simulink library "momentumVelocityControl_lib"  (R2020b)
settings: Solver=VariableStepAuto  StartTime=0.0  StopTime=10.0  RelTol=1e-3
undefined symbols (not defined in the file): bVectorConstraints, Config, ConstraintsMatrix, ROBOT_DOF, Sat
settings Model: Creator=csartore  LastModifiedBy=csartore

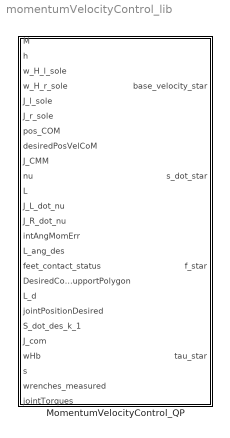
== system momentumVelocityControl_lib ==
  MomentumVelocityControl_QP : Subsystem

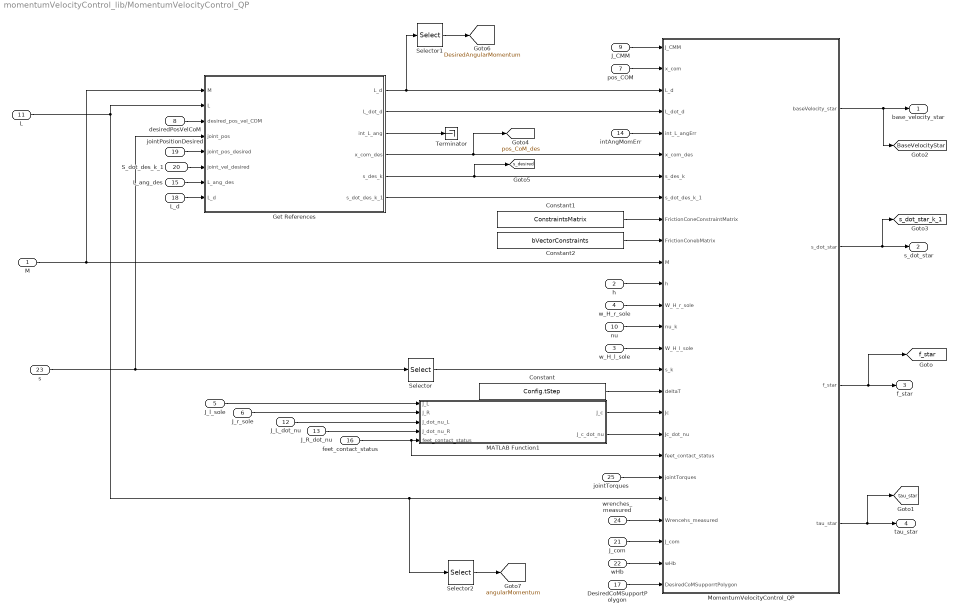
== system momentumVelocityControl_lib/MomentumVelocityControl_QP ==
  M : Inport
  h : Inport  Port=2
  w_H_l_sole : Inport  Port=3
  w_H_r_sole : Inport  Port=4
  J_l_sole : Inport  Port=5
  J_r_sole : Inport  Port=6
  pos_COM : Inport  Port=7
  desiredPosVelCoM : Inport  Port=8
  J_CMM : Inport  Port=9
  nu : Inport  Port=10
  L : Inport  Port=11
  J_L_dot_nu : Inport  Port=12
  J_R_dot_nu : Inport  Port=13
  intAngMomErr : Inport  Port=14
  L_ang_des : Inport  Port=15
  feet_contact_status : Inport  Port=16
  DesiredCoMSupportPolygon : Inport  Port=17
  L_d : Inport  Port=18
  jointPositionDesired : Inport  Port=19
  S_dot_des_k_1 : Inport  Port=20
  J_com : Inport  Port=21
  wHb : Inport  Port=22
  s : Inport  Port=23
  wrenches_measured : Inport  Port=24
  jointTorques : Inport  Port=25
  Constant : Constant  Value=Config.tStep
  Constant1 : Constant  Value=ConstraintsMatrix
  Constant2 : Constant  Value=bVectorConstraints
  Get References : MATLAB Function  TreatAsAtomicUnit=on
  MATLAB Function1 : MATLAB Function  TreatAsAtomicUnit=on
  MomentumVelocityControl_QP : Subsystem
  Selector : Selector  InputPortWidth=ROBOT_DOF  IndexOptions=Index vector (dialog)  Indices=[1:ROBOT_DOF]  OutputSizes=1
  Selector1 : Selector  InputPortWidth=6  IndexOptions=Index vector (dialog)  Indices=[4:6]  OutputSizes=1
  Selector2 : Selector  InputPortWidth=6  IndexOptions=Index vector (dialog)  Indices=[4:6]  OutputSizes=1
  Terminator : Terminator
  base_velocity_star : Outport
  s_dot_star : Outport  Port=2
  f_star : Outport  Port=3
  tau_star : Outport  Port=4
  tag scope: BaseVelocityStar=global, DesiredAngularMomentum=global, angularMomentum=global, f_star=global, pos_CoM_des=global, s_desired=global, s_dot_star_k_1=global, tau_star=global
  wires:
  DesiredCoMSupportPolygon/1 -> MomentumVelocityControl_QP/26(DesiredCoMSupporrtPolygon)
  Get References/6(s_dot_des_k_1) -> MomentumVelocityControl_QP/8(s_dot_des_k_1)
  Selector2/1 -> [angularMomentum]
  Selector1/1 -> [DesiredAngularMomentum]
  Selector/1 -> MomentumVelocityControl_QP/16(s_k)
  h/1 -> MomentumVelocityControl_QP/12(h)
  L/1 -> MomentumVelocityControl_QP/22(L), Selector2/1, Get References/2(L)
  J_CMM/1 -> MomentumVelocityControl_QP/1(J_CMM)
  MATLAB Function1/2(J_c_dot_nu) -> MomentumVelocityControl_QP/19(Jc_dot_nu)
  intAngMomErr/1 -> MomentumVelocityControl_QP/5(int_L_angErr)
  MomentumVelocityControl_QP/2(s_dot_star) -> [s_dot_star_k_1], s_dot_star/1
  MomentumVelocityControl_QP/1(baseVelocity_star) -> [BaseVelocityStar], base_velocity_star/1
  MATLAB Function1/1(J_c) -> MomentumVelocityControl_QP/18(Jc)
  nu/1 -> MomentumVelocityControl_QP/14(nu_k)
  feet_contact_status/1 -> MATLAB Function1/5(feet_contact_status), MomentumVelocityControl_QP/20(feet_contact_status)
  MomentumVelocityControl_QP/4(tau_star) -> [tau_star], tau_star/1
  L_ang_des/1 -> Get References/7(L_ang_des)
  Get References/5(s_des_k) -> MomentumVelocityControl_QP/7(s_des_k), [s_desired]
  pos_COM/1 -> MomentumVelocityControl_QP/2(x_com)
  w_H_r_sole/1 -> MomentumVelocityControl_QP/13(W_H_r_sole)
  w_H_l_sole/1 -> MomentumVelocityControl_QP/15(W_H_l_sole)
  J_r_sole/1 -> MATLAB Function1/2(J_R)
  Get References/2(L_dot_d) -> MomentumVelocityControl_QP/4(L_dot_d)
  jointPositionDesired/1 -> Get References/5(joint_pos_desired)
  J_R_dot_nu/1 -> MATLAB Function1/4(J_dot_nu_R)
  s/1 -> Selector/1, Get References/4(joint_pos)
  jointTorques/1 -> MomentumVelocityControl_QP/21(jointTorques)
  J_L_dot_nu/1 -> MATLAB Function1/3(J_dot_nu_L)
  wHb/1 -> MomentumVelocityControl_QP/25(wHb)
  wrenches_measured/1 -> MomentumVelocityControl_QP/23(Wrencehs_measured)
  Constant1/1 -> MomentumVelocityControl_QP/9(FrictionConeConstraintMatrix)
  M/1 -> MomentumVelocityControl_QP/11(M), Get References/1(M)
  MomentumVelocityControl_QP/3(f_star) -> [f_star], f_star/1
  Constant/1 -> MomentumVelocityControl_QP/17("deltaT ")
  Constant2/1 -> MomentumVelocityControl_QP/10(FrictionConebMatrix)
  Get References/4(x_com_des) -> MomentumVelocityControl_QP/6(x_com_des), [pos_CoM_des]
  J_l_sole/1 -> MATLAB Function1/1(J_L)
  Get References/1(L_d) -> Selector1/1, MomentumVelocityControl_QP/3(L_d)
  Get References/3(int_L_ang) -> Terminator/1
  J_com/1 -> MomentumVelocityControl_QP/24(J_com)
  desiredPosVelCoM/1 -> Get References/3(desired_pos_vel_COM)
  L_d/1 -> Get References/8("L_d ")
  S_dot_des_k_1/1 -> Get References/6(joint_vel_desired)

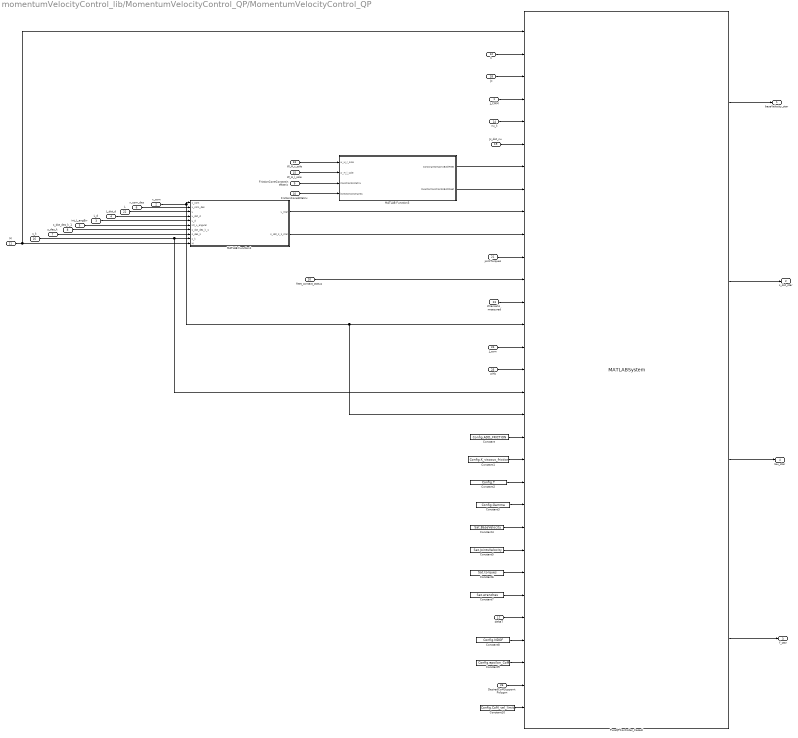
== system momentumVelocityControl_lib/MomentumVelocityControl_QP/MomentumVelocityControl_QP ==
  J_CMM : Inport
  x_com : Inport  Port=2
  L_d : Inport  Port=3
  L_dot_d : Inport  Port=4
  int_L_angErr : Inport  Port=5
  x_com_des : Inport  Port=6
  s_des_k : Inport  Port=7
  s_dot_des_k_1 : Inport  Port=8
  FrictionConeConstraintMatrix : Inport  Port=9
  FrictionConebMatrix : Inport  Port=10
  M : Inport  Port=11
  h : Inport  Port=12
  W_H_r_sole : Inport  Port=13
  nu_k : Inport  Port=14
  W_H_l_sole : Inport  Port=15
  s_k : Inport  Port=16
  "deltaT " : Inport  Port=17
  Jc : Inport  Port=18
  Jc_dot_nu : Inport  Port=19
  feet_contact_status : Inport  Port=20
  jointTorques : Inport  Port=21
  L : Inport  Port=22
  Wrencehs_measured : Inport  Port=23
  J_com : Inport  Port=24
  wHb : Inport  Port=25
  DesiredCoMSupporrtPolygon : Inport  Port=26
  Constant : Constant  Value=Config.ADD_FRICTION
  Constant1 : Constant  Value=Config.K_viscous_friction
  Constant10 : Constant  Value=Config.CoM_vel_limits  VectorParams1D=off
  Constant2 : Constant  Value=Config.T
  Constant3 : Constant  Value=Config.Gamma
  Constant4 : Constant  Value=Sat.BaseVelocity  VectorParams1D=off
  Constant5 : Constant  Value=Sat.JointsVelocity  VectorParams1D=off
  Constant6 : Constant  Value=Sat.torques  VectorParams1D=off
  Constant7 : Constant  Value=Sat.wrenches  VectorParams1D=off
  Constant8 : Constant  Value=Config.NDOF  VectorParams1D=off
  Constant9 : Constant  Value=Config.epsilon_CoM  VectorParams1D=off
  MATLAB Function1 : MATLAB Function  TreatAsAtomicUnit=on
  MATLAB Function3 : MATLAB Function  TreatAsAtomicUnit=on
  PureQPController_Casadi : MATLABSystem  System=casadi_block  SimulateUsing=Interpreted execution
      mask Type: casadi_block
      mask Display:
      | disp('casadi_block');
      | port_label('input',1,'M');
      | port_label('input',2,'h');
      | port_label('input',3,'Jc');
      | port_label('input',4,'Jcmm');
      | port_label('input',5,'nu_k');
      | port_label('input',6,'Jc_dot_nu');
      | port_label('input',7,'C_friction');
      | port_label('input',8,'b_friction');
      | port_label('input',9,'H_star');
      | port_label('input',10,'s_dot_star');
      | port_label('input',11,'tau_meas');
      | port_label('input',12,'contact_status');
      | port_label('input',13,'f_meas');
      | port_label('input',14,'x_com');
      | port_label('input',15,'J_com');
      | port_label('input',16,'w_H_b');
      | port_label('input',17,'s');
      | port_label('input',18,'CoM_measured');
      | port_label('input',19,'ADD_FRICTION');
      | port_label('input',20,'K_viscous_friction');
      | port_label('input',21,'T');
      | port_label('input',22,'Gamma');
      | port_label('input',23,'baseVelocitySat');
      | port_label('input',24,'jointsVelocitySat');
      | port_label('input',25,'torqueSat');
      | port_label('input',26,'wrenchesSat');
      | port_label('input',27,'tStep');
      | port_label('input',28,'NDOF');
      | port_label('input',29,'epsilon_CoM');
      | port_label('input',30,'CoM_limits');
      | port_label('input',31,'CoM_vel_limits');
      | port_label('output',1,'v_b_star');
      | port_label('output',2,'s_dot_k_1_star');
      | port_label('output',3,'tau_star');
      | port_label('output',4,'f_star');
  baseVelocity_star : Outport
  s_dot_star : Outport  Port=2
  f_star : Outport  Port=3
  tau_star : Outport  Port=4
  wires:
  PureQPController_Casadi/4 -> f_star/1
  PureQPController_Casadi/1 -> baseVelocity_star/1
  PureQPController_Casadi/3 -> tau_star/1
  PureQPController_Casadi/2 -> s_dot_star/1
  Constant10/1 -> PureQPController_Casadi/31
  DesiredCoMSupporrtPolygon/1 -> PureQPController_Casadi/30
  Constant9/1 -> PureQPController_Casadi/29
  Constant8/1 -> PureQPController_Casadi/28
  "deltaT "/1 -> PureQPController_Casadi/27
  Constant7/1 -> PureQPController_Casadi/26
  Constant6/1 -> PureQPController_Casadi/25
  Constant5/1 -> PureQPController_Casadi/24
  Constant4/1 -> PureQPController_Casadi/23
  Constant3/1 -> PureQPController_Casadi/22
  Constant2/1 -> PureQPController_Casadi/21
  Constant1/1 -> PureQPController_Casadi/20
  Constant/1 -> PureQPController_Casadi/19
  jointTorques/1 -> PureQPController_Casadi/11
  MATLAB Function1/1(L_star) -> PureQPController_Casadi/9
  MATLAB Function1/2(s_dot_k_1_star) -> PureQPController_Casadi/10
  MATLAB Function3/1(ConstraintsMatrixBothFeet) -> PureQPController_Casadi/7
  MATLAB Function3/2(bVectorConstraintsBothFeet) -> PureQPController_Casadi/8
  W_H_r_sole/1 -> MATLAB Function3/1(w_H_r_sole)
  W_H_l_sole/1 -> MATLAB Function3/2(w_H_l_sole)
  x_com/1 -> MATLAB Function1/1(x_com), PureQPController_Casadi/14, PureQPController_Casadi/18
  x_com_des/1 -> MATLAB Function1/2(x_com_des)
  L/1 -> MATLAB Function1/3(L)
  L_dot_d/1 -> MATLAB Function1/4(L_dot_d)
  L_d/1 -> MATLAB Function1/5(L_d)
  int_L_angErr/1 -> MATLAB Function1/6(int_L_angular)
  s_des_k/1 -> MATLAB Function1/8(s_des_k)
  s_dot_des_k_1/1 -> MATLAB Function1/7(s_dot_des_k_1)
  M/1 -> MATLAB Function1/10(M), PureQPController_Casadi/1
  feet_contact_status/1 -> PureQPController_Casadi/12
  Jc/1 -> PureQPController_Casadi/3
  J_CMM/1 -> PureQPController_Casadi/4
  nu_k/1 -> PureQPController_Casadi/5
  Jc_dot_nu/1 -> PureQPController_Casadi/6
  h/1 -> PureQPController_Casadi/2
  FrictionConeConstraintMatrix/1 -> MATLAB Function3/3(ConstraintsMatrix)
  FrictionConebMatrix/1 -> MATLAB Function3/4(bVectorConstraints)
  Wrencehs_measured/1 -> PureQPController_Casadi/13
  J_com/1 -> PureQPController_Casadi/15
  wHb/1 -> PureQPController_Casadi/16
  s_k/1 -> PureQPController_Casadi/17, MATLAB Function1/9(s_k)

== matlab function momentumVelocityControl_lib/MomentumVelocityControl_QP/Get References ==
  data: M input; L input; L_d output; L_dot_d output; desired_pos_vel_COM input; joint_pos input; int_L_ang output; x_com_des output; s_des_k output; s_dot_des_k_1 output; joint_pos_desired input; joint_vel_desired input; L_ang_des input; L_d input
function [L_d, L_dot_d, int_L_ang,x_com_des, s_des_k,s_dot_des_k_1]= ComputeReferencesFCN(M,L,desired_pos_vel_COM, joint_pos, joint_pos_desired,joint_vel_desired, L_ang_des,L_d)
[L_d, L_dot_d, int_L_ang,x_com_des, s_des_k,s_dot_des_k_1]= ComputeReferencesController(M,L,desired_pos_vel_COM, joint_pos, joint_pos_desired,joint_vel_desired, L_ang_des,L_d);

end

== matlab function momentumVelocityControl_lib/MomentumVelocityControl_QP/MATLAB Function1 ==
  data: J_L input; J_c output; J_R input; J_dot_nu_L input; J_dot_nu_R input; J_c_dot_nu output; feet_contact_status input
function [J_c,J_c_dot_nu] = ComputeContactJacobianWithFeetContact(J_L,J_R,J_dot_nu_L, J_dot_nu_R, feet_contact_status)


[J_c,J_c_dot_nu] = ComputeContactJacobianWithFeetContactFCN(J_L,J_R,J_dot_nu_L, J_dot_nu_R, feet_contact_status);

end

== matlab function momentumVelocityControl_lib/MomentumVelocityControl_QP/MomentumVelocityControl_QP/MATLAB Function1 ==
  data: x_com input; L_star output; x_com_des input; L input; L_dot_d input; L_d input; int_L_angular input; s_dot_des_k_1 input; s_des_k input; s_k input; M input; s_dot_k_1_star output; Gains parameter
function [L_star, s_dot_k_1_star] = ComputeReferencesFCN(x_com, x_com_des, L, L_dot_d, L_d, int_L_angular, s_dot_des_k_1, s_des_k, s_k, M,Gains) 

[L_star, L_dot_star, s_dot_k_1_star] = ComputeReferences(x_com, x_com_des, L, L_dot_d, L_d, int_L_angular, s_dot_des_k_1, s_des_k, s_k, M(1,1),Gains); 

end

== matlab function momentumVelocityControl_lib/MomentumVelocityControl_QP/MomentumVelocityControl_QP/MATLAB Function3 ==
  data: w_H_r_sole input; ConstraintsMatrixBothFeet output; w_H_l_sole input; ConstraintsMatrix input; bVectorConstraints input; bVectorConstraintsBothFeet output
function [ConstraintsMatrixBothFeet,bVectorConstraintsBothFeet] = ComputeConstraintMatrix(w_H_r_sole,w_H_l_sole,ConstraintsMatrix,bVectorConstraints)
w_R_r_sole                 = w_H_r_sole(1:3,1:3);
w_R_l_sole                 = w_H_l_sole(1:3,1:3);
ConstraintMatrixLeftFoot   = ConstraintsMatrix * blkdiag(w_R_l_sole', w_R_l_sole');
ConstraintMatrixRightFoot  = ConstraintsMatrix * blkdiag(w_R_r_sole', w_R_r_sole');
ConstraintsMatrixBothFeet  = blkdiag(ConstraintMatrixLeftFoot, ConstraintMatrixRightFoot);
bVectorConstraintsBothFeet = [bVectorConstraints; bVectorConstraints];
end
